simulink model "splitting_power_demand"  (R2020a)
settings: Solver=VariableStepAuto  StartTime=0.0  StopTime=100  RelTol=1e-3
libraries: simulink x1
settings Model: Creator=sateeshk  LastModifiedBy=sateeshk

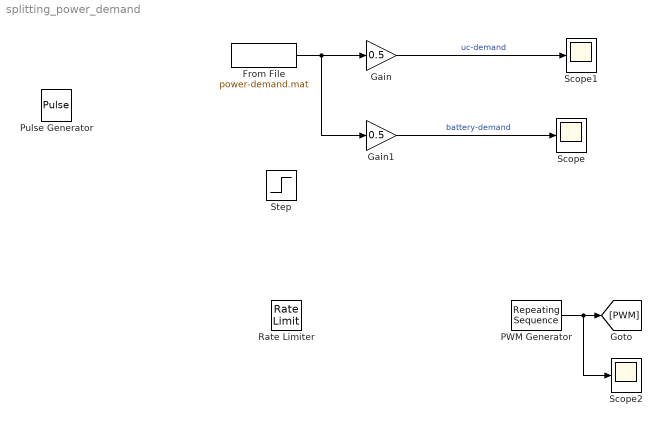
== system splitting_power_demand ==
  From File : FromFile  FileName=power-demand.mat  SampleTime=0
  Gain : Gain  Gain=0.5
  Gain1 : Gain  Gain=0.5
  PWM Generator : simulink/Sources/Repeating Sequence  rep_seq_t="[0 1/4*0.0001  2/4*0.0001  3/4*0.0001  0.0001]"  rep_seq_y=[0 1 0 -1 0]
  Pulse Generator : DiscretePulseGenerator  PulseType=Time based  Amplitude=400  Period=10  PulseWidth=50
  Rate Limiter : RateLimiter  RisingSlewLimit=300  FallingSlewLimit=-300  SampleTimeMode=inherited
  Scope : Scope
  Scope1 : Scope
  Scope2 : Scope
  Step : Step  After=100  SampleTime=0
  wires:
  Gain/1 -> Scope1/1  "uc-demand"
  Gain1/1 -> Scope/1  "battery-demand"
  PWM Generator/1 -> Scope2/1, [PWM]
  From File/1 -> Gain1/1, Gain/1
